simulink model "step4_EvapCompCondHarness"  (R2023a)
settings: Solver=VariableStepAuto  StartTime=0.0  StopTime=36000  RelTol=1e-3  AbsTol=1e-3
model workspace (MATLAB code in the model file):
  | evapCompCondParams;
undefined symbols (not defined in the file): a_x_cond, mdot_air_cond, T0
libraries: fl_lib x43, nesl_utility x9, SimscapeFluids_lib x4
CloseFcn:
  | try,close(h1_step4_EvapCompCondHarness),end
  | clear h1_step4_EvapCompCondHarness
  | try,close(h2_step4_EvapCompCondHarness),end
  | clear h2_step4_EvapCompCondHarness
  | try,close(h3_step4_EvapCompCondHarness),end
  | clear h3_step4_EvapCompCondHarness
  | try,close(h4_step4_EvapCompCondHarness),end
  | clear h4_step4_EvapCompCondHarness
  | 
  | 
  | clear simlog_step4_EvapCompCondHarness
  | clear logsout_step4_EvapCompCondHarness
settings Model: Creator=emcgarri  LastModifiedBy=esmithzb
settings SolverCC: AutoScaleAbsTol=off  AlgebraicLoopSolver=TrustRegion  DecoupledContinuousIntegration=on  MinimalZcImpactIntegration=on  MaxZcPerStep=1
settings DataIOCC: MaxDataPoints=10000  SignalLoggingName=logsout_step4_EvapCompCondHarness
settings OptimizationCC: ReuseModelBlockBuffer=off
settings DebuggingCC: UnconnectedInputMsg=warning  UnconnectedOutputMsg=warning  UnconnectedLineMsg=warning  SymbolicDimsDataTypeCodeGenerationDiagnostic=none
settings ModelReferenceCC: EnableRefExpFcnMdlSchedulingChecks=on
settings SFSimCC: CustomCodeUndefinedFunction=UseInterfaceOnly
settings RTWCC: DLArmComputeVersion=19.05
settings SimscapeCC: SimscapeLogType=all  SimscapeLogSimulationStatistics=on  SimscapeLogOpenViewer=on  SimscapeLogName=simlog_step4_EvapCompCondHarness  SimscapeLogDataHistory=10000

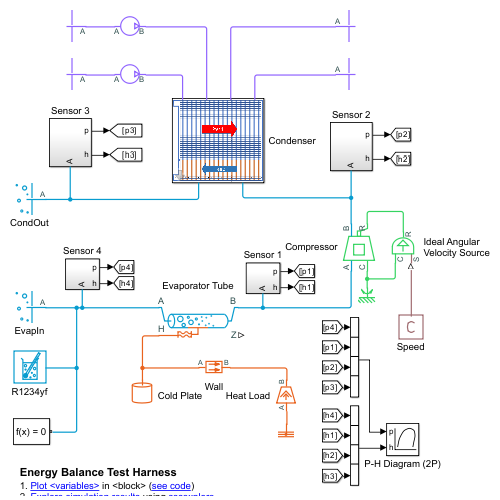
[thumbnail: Simulink's stored preview of the top-level diagram]
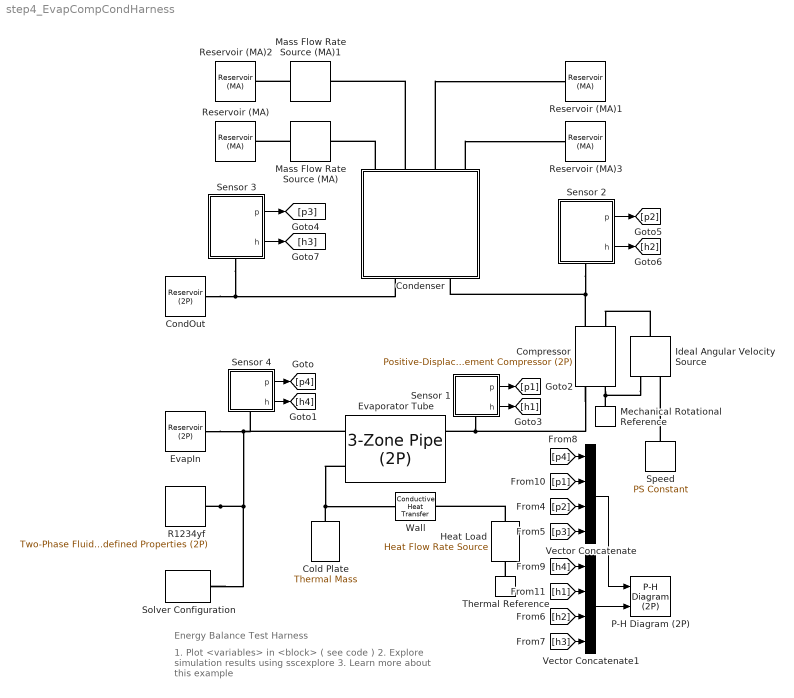
== system step4_EvapCompCondHarness ==
  note: Energy Balance Test Harness
  note: 1. Plot <variables> in <block> ( see code )
      | 2. Explore simulation results using sscexplore
      | 3. Learn more about this example
  Cold Plate : fl_lib/Thermal/Thermal Elements/Thermal Mass  mass_type=foundation.enum.constant_variable.constant  mass=m_plate kg  sp_heat=cp_plate J/(K*kg)  mass_min=1e-6 kg  num_ports=foundation.enum.numPorts2.one  m_specify=off  m_priority=High  m=1 kg  m_nominal_specify=off  m_nominal_unit=kg  m_nominal_value=1  T_specify=on  T_priority=High  T=T0 K  T_nominal_specify=off  T_nominal_unit=K  T_nominal_value=1  Q_specify=off  Q_priority=None  Q=0 W  Q_nominal_specify=off  Q_nominal_unit=W  Q_nominal_value=1
  Compressor : SimscapeFluids_lib/Two-Phase Fluid/Fluid Machines/Positive-Displacement Compressor (2P)  dispSpec=fluids.two_phase_fluid.fluid_machines.enum.DisplacementSpecification.FlowSpeed  v_disp=130 cm^3/rev  mdot_nom=mdot_comp kg/s  omega_nom=N_comp rpm  efficiencySpec=fluids.two_phase_fluid.fluid_machines.enum.VolumetricEfficiencyParameterization.Analytical  eta_nom=eta_v  pr_TLU=[2, 4, 6, 8]  omega_TLU=[800, 1500, 2800, 3300, 4000] rpm  eta_TLU=[.95, .9, .85, .8, .75; .925, .875, .825, .775, .725; .875, .825, .775, .725, .675; .75, .7, .65, .6, .55]  nominalSpec=fluids.two_phase_fluid.fluid_machines.enum.NominalConditionsSpecification.NominalEffandPR  pr_nom=pr_nom  p_in_nom=p_nom_in kPa  T_in_nom=T_nom_in K  T_evap_nom=373.15 K  T_cond_nom=398.15 K  delta_T_nom=10 deltaK  n=gamma1234yf  mechanical_efficiency=eta_m  area_A=a_evap cm^2  area_B=a_cond cm^2  VaporCheck=simscape.enum.assert.action.warn
      settings: InternalSimscapePortConfiguration="{\"Bottom\":[],\"Left\":[{\"id\":\"A\",\"label\":\"A\",\"type\":\"foundation.two_phase_fluid.two_phase_fluid\"},{\"id\":\"C\",\"label\":\"C\",\"type\":\"foundation.mechanical.rotational.rotational\"}],\"Right\":[{\"id\":\"B\",\"label\":\"B\",\"type\":\"foundation.two_phase_fluid.two_phase_fluid\"},{\"id\":\"R\",\"label\":\"R\",\"type\":\"foundation.mechanical.rotational.rotational\"}],\"Top\":[]}"
  CondOut : fl_lib/Two-Phase Fluid/Elements/Reservoir (2P)  pressure_spec=foundation.enum.ReservoirPressureSpec2P.Specified  reservoir_pressure=p0_cond kPa  reservoir_condensing_temperature=373.15 K  reservoir_evaporating_temperature=373.15 K  energy_spec=foundation.enum.ReservoirEnergySpec2P.Enthalpy  reservoir_temperature=293.15 K  reservoir_quality=0.5  reservoir_void_fraction=0.5  reservoir_enthalpy=h0_cond kJ/kg  reservoir_internal_energy=1500 kJ/kg  reservoir_subcooling=5 deltaK  reservoir_superheating=5 deltaK  area_A=a_cond cm^2
  Condenser : Subsystem  ReferencedSubsystem=Condenser_2Pass  p_init=p0_cond kPa  IC_spec=Specific Enthalpy  h_init=h0_cond kJ/kg  x_init=x0  energy_spec=foundation.enum.energy_spec.enthalpy
  EvapIn : fl_lib/Two-Phase Fluid/Elements/Reservoir (2P)  pressure_spec=foundation.enum.ReservoirPressureSpec2P.Specified  reservoir_pressure=p0_evap kPa  reservoir_condensing_temperature=373.15 K  reservoir_evaporating_temperature=373.15 K  energy_spec=foundation.enum.ReservoirEnergySpec2P.Enthalpy  reservoir_temperature=293.15 K  reservoir_quality=0.5  reservoir_void_fraction=0.5  reservoir_enthalpy=h0_evap kJ/kg  reservoir_internal_energy=1500 kJ/kg  reservoir_subcooling=5 deltaK  reservoir_superheating=5 deltaK  area_A=a_evap cm^2
  Evaporator Tube : SimscapeFluids_lib/Two-Phase Fluid/Pipes & Fittings/3-Zone Pipe (2P)  length=l_evap m  area=a_evap cm^2  Dh=d_evap cm  length_add=0 m  roughness=15e-6 m  Re_lam=2000  Re_tur=4000  shape_factor=64  hc_ext=inf W/(m^2*K)  wall_thickness=1 mm  k_wall=k_plate W/(m*K)  c_wall=cp_plate J/(K*kg)  rho_wall=rho_plate kg/m^3  fin_ratio_ext=0  eta_fin_ext=0.5  fin_ratio_int=0  eta_fin_int=0.5  heat_coeff_spec=fluids.two_phase_fluid.pipes_fittings.enum.HeatCoeffSpec.GnielinskiCavalliniZecchin  colburn_coeff_liq=[.023, .8, .33]  colburn_coeff_mix=[.05, .8, .33]  colburn_coeff_vap=[.023, .8, .33]  Nu_lam=3.66  energy_spec=foundation.enum.energy_spec.enthalpy  p_init=p0_evap kPa  T_init=293.15 K  x_init=0.5  alpha_init=0.5  h_init=h0_evap kJ/kg  u_init=1500 kJ/kg
      settings: InternalSimscapePortConfiguration="{\"Bottom\":[],\"Left\":[{\"id\":\"A\",\"label\":\"A\",\"type\":\"foundation.two_phase_fluid.two_phase_fluid\"},{\"id\":\"H\",\"label\":\"H\",\"type\":\"foundation.thermal.thermal\"}],\"Right\":[{\"id\":\"B\",\"label\":\"B\",\"type\":\"foundation.two_phase_fluid.two_phase_fluid\"},{\"id\":\"Z\",\"label\":\"Z\",\"type\":\"output\"}],\"Top\":[]}"
  Heat Load : fl_lib/Thermal/Thermal Sources/Heat Flow Rate Source  heat_flow=1 kW
      settings: InternalSimscapePortConfiguration="{\"Bottom\":[],\"Left\":[{\"id\":\"B\",\"label\":\"B\",\"type\":\"foundation.thermal.thermal\"}],\"Right\":[{\"id\":\"A\",\"label\":\"A\",\"type\":\"foundation.thermal.thermal\"}],\"Top\":[]}"
  Ideal Angular Velocity Source : fl_lib/Mechanical/Mechanical Sources/Ideal Angular Velocity Source
  Mass Flow Rate Source (MA) : fl_lib/Moist Air/Sources/Mass Flow Rate Source (MA)  power_spec=foundation.enum.power_spec.none  mass_flow=mdot_air_cond(2) kg/s  area_A=a_x_cond(2) m^2  area_B=a_x_cond(2) m^2
      settings: InternalSimscapePortConfiguration="{\"Bottom\":[],\"Left\":[{\"id\":\"A\",\"label\":\"A\",\"type\":\"foundation.moist_air.moist_air\"}],\"Right\":[{\"id\":\"B\",\"label\":\"B\",\"type\":\"foundation.moist_air.moist_air\"}],\"Top\":[]}"
  Mass Flow Rate Source (MA)1 : fl_lib/Moist Air/Sources/Mass Flow Rate Source (MA)  power_spec=foundation.enum.power_spec.none  mass_flow=mdot_air_cond(1) kg/s  area_A=a_x_cond(1) cm^2  area_B=a_x_cond(1) cm^2
      settings: InternalSimscapePortConfiguration="{\"Bottom\":[],\"Left\":[{\"id\":\"A\",\"label\":\"A\",\"type\":\"foundation.moist_air.moist_air\"}],\"Right\":[{\"id\":\"B\",\"label\":\"B\",\"type\":\"foundation.moist_air.moist_air\"}],\"Top\":[]}"
  Mechanical Rotational Reference : fl_lib/Mechanical/Rotational Elements/Mechanical Rotational Reference
  P-H Diagram (2P) : SimscapeFluids_lib/Two-Phase Fluid/Utilities/P-H Diagram (2P)
  R1234yf : SimscapeFluids_lib/Two-Phase Fluid/Utilities/Two-Phase Fluid Predefined Properties (2P)  fluid=fluids.two_phase_fluid.utilities.enum.Fluid.R1234yf  p_atm=0.101325 MPa  properties_range_check=simscape.enum.assert.action.error  q_rev=0.01 Pa
  Reservoir (MA) : fl_lib/Moist Air/Elements/Reservoir (MA)  pressure_spec=foundation.enum.pressure_spec.atmospheric  reservoir_pressure=0.101325 MPa  temperature_spec=foundation.enum.temperature_spec.specified  reservoir_temperature=T_air_cond degC  moisture_spec=foundation.enum.moisture_spec.relative_humidity  reservoir_RH=0.5  reservoir_x_w=0.01  reservoir_y_w=0.01  reservoir_HR=0.01  reservoir_Tw=287 K  trace_gas_spec=foundation.enum.trace_gas_spec.mass_fraction  reservoir_x_g=0.00  reservoir_y_g=0.001  RH_ws=1  area_A=a_x_cond(2) cm^2
  Reservoir (MA)1 : fl_lib/Moist Air/Elements/Reservoir (MA)  pressure_spec=foundation.enum.pressure_spec.atmospheric  reservoir_pressure=0.101325 MPa  temperature_spec=foundation.enum.temperature_spec.atmospheric  reservoir_temperature=293.15 K  moisture_spec=foundation.enum.moisture_spec.relative_humidity  reservoir_RH=0.5  reservoir_x_w=0.01  reservoir_y_w=0.01  reservoir_HR=0.01  reservoir_Tw=287 K  trace_gas_spec=foundation.enum.trace_gas_spec.mass_fraction  reservoir_x_g=0.001  reservoir_y_g=0.001  RH_ws=1  area_A=a_x_cond(2) cm^2
  Reservoir (MA)2 : fl_lib/Moist Air/Elements/Reservoir (MA)  pressure_spec=foundation.enum.pressure_spec.atmospheric  reservoir_pressure=0.101325 MPa  temperature_spec=foundation.enum.temperature_spec.specified  reservoir_temperature=T_air_cond degC  moisture_spec=foundation.enum.moisture_spec.relative_humidity  reservoir_RH=0.5  reservoir_x_w=0.01  reservoir_y_w=0.01  reservoir_HR=0.01  reservoir_Tw=287 K  trace_gas_spec=foundation.enum.trace_gas_spec.mass_fraction  reservoir_x_g=0.00  reservoir_y_g=0.001  RH_ws=1  area_A=a_x_cond(1) cm^2
  Reservoir (MA)3 : fl_lib/Moist Air/Elements/Reservoir (MA)  pressure_spec=foundation.enum.pressure_spec.atmospheric  reservoir_pressure=0.101325 MPa  temperature_spec=foundation.enum.temperature_spec.atmospheric  reservoir_temperature=293.15 K  moisture_spec=foundation.enum.moisture_spec.relative_humidity  reservoir_RH=0.5  reservoir_x_w=0.01  reservoir_y_w=0.01  reservoir_HR=0.01  reservoir_Tw=287 K  trace_gas_spec=foundation.enum.trace_gas_spec.mass_fraction  reservoir_x_g=0.001  reservoir_y_g=0.001  RH_ws=1  area_A=a_x_cond(1) cm^2
  Sensor 1 : Subsystem
      settings: PortSchema="{\"entries\":[{\"content\":{\"sides\":[{\"content\":{\"connectorIds\":[]},\"type\":\"ConnectorPlacement.EquallySpacedRectSide\",\"uuid\":\"09a2fde7-9514-415f-ad1a-2358fbc90122\"},{\"content\":{\"connectorIds\":[\"Out1\",\"Out2\"],\"side\":\"RIGHT\"},\"type\":\"ConnectorPlacement.EquallySpacedRectSide\",\"uuid\":\"1a58e595-65c2-481f-a4c6-044a1080df7a\"},{\"content\":{\"connectorIds\":[],\"side\":\"TOP\"},\"type\":\"ConnectorPlacement.EquallySpacedRectSide\",\"uuid\":\"e920d07f-3316-48c2-b5dc-69759bfb2eca\"},{\"content\":{\"connectorIds\":[\"RConn1\"],\"side\":\"BOTTOM\"},\"type\":\"ConnectorPlacement.EquallySpacedRectSide\",\"uuid\":\"ceb1a63b-e9f5-46e4-b72f-4e0e29463411\"}]},\"type\":\"ConnectorPlacement.EquallySpacedConnector\",\"uuid\":\"10759918-f7d5-4efa-b411-b89b519c736f\"}],\"packageUris\":[\"http://schema.mathworks.com/mf0/Connector/R2020b\"],\"version\":\"1.0\"}"
  Sensor 2 : Subsystem
      settings: PortSchema="{\"entries\":[{\"content\":{\"sides\":[{\"content\":{\"connectorIds\":[]},\"type\":\"ConnectorPlacement.EquallySpacedRectSide\",\"uuid\":\"09a2fde7-9514-415f-ad1a-2358fbc90122\"},{\"content\":{\"connectorIds\":[\"Out1\",\"Out2\"],\"side\":\"RIGHT\"},\"type\":\"ConnectorPlacement.EquallySpacedRectSide\",\"uuid\":\"1a58e595-65c2-481f-a4c6-044a1080df7a\"},{\"content\":{\"connectorIds\":[],\"side\":\"TOP\"},\"type\":\"ConnectorPlacement.EquallySpacedRectSide\",\"uuid\":\"e920d07f-3316-48c2-b5dc-69759bfb2eca\"},{\"content\":{\"connectorIds\":[\"RConn1\"],\"side\":\"BOTTOM\"},\"type\":\"ConnectorPlacement.EquallySpacedRectSide\",\"uuid\":\"ceb1a63b-e9f5-46e4-b72f-4e0e29463411\"}]},\"type\":\"ConnectorPlacement.EquallySpacedConnector\",\"uuid\":\"10759918-f7d5-4efa-b411-b89b519c736f\"}],\"packageUris\":[\"http://schema.mathworks.com/mf0/Connector/R2020b\"],\"version\":\"1.0\"}"
  Sensor 3 : Subsystem
      settings: PortSchema="{\"entries\":[{\"content\":{\"sides\":[{\"content\":{\"connectorIds\":[]},\"type\":\"ConnectorPlacement.EquallySpacedRectSide\",\"uuid\":\"09a2fde7-9514-415f-ad1a-2358fbc90122\"},{\"content\":{\"connectorIds\":[\"Out1\",\"Out2\"],\"side\":\"RIGHT\"},\"type\":\"ConnectorPlacement.EquallySpacedRectSide\",\"uuid\":\"1a58e595-65c2-481f-a4c6-044a1080df7a\"},{\"content\":{\"connectorIds\":[],\"side\":\"TOP\"},\"type\":\"ConnectorPlacement.EquallySpacedRectSide\",\"uuid\":\"e920d07f-3316-48c2-b5dc-69759bfb2eca\"},{\"content\":{\"connectorIds\":[\"RConn1\"],\"side\":\"BOTTOM\"},\"type\":\"ConnectorPlacement.EquallySpacedRectSide\",\"uuid\":\"ceb1a63b-e9f5-46e4-b72f-4e0e29463411\"}]},\"type\":\"ConnectorPlacement.EquallySpacedConnector\",\"uuid\":\"10759918-f7d5-4efa-b411-b89b519c736f\"}],\"packageUris\":[\"http://schema.mathworks.com/mf0/Connector/R2020b\"],\"version\":\"1.0\"}"
  Sensor 4 : Subsystem
      settings: PortSchema="{\"entries\":[{\"content\":{\"sides\":[{\"content\":{\"connectorIds\":[]},\"type\":\"ConnectorPlacement.EquallySpacedRectSide\",\"uuid\":\"09a2fde7-9514-415f-ad1a-2358fbc90122\"},{\"content\":{\"connectorIds\":[\"Out1\",\"Out2\"],\"side\":\"RIGHT\"},\"type\":\"ConnectorPlacement.EquallySpacedRectSide\",\"uuid\":\"1a58e595-65c2-481f-a4c6-044a1080df7a\"},{\"content\":{\"connectorIds\":[],\"side\":\"TOP\"},\"type\":\"ConnectorPlacement.EquallySpacedRectSide\",\"uuid\":\"e920d07f-3316-48c2-b5dc-69759bfb2eca\"},{\"content\":{\"connectorIds\":[\"RConn1\"],\"side\":\"BOTTOM\"},\"type\":\"ConnectorPlacement.EquallySpacedRectSide\",\"uuid\":\"ceb1a63b-e9f5-46e4-b72f-4e0e29463411\"}]},\"type\":\"ConnectorPlacement.EquallySpacedConnector\",\"uuid\":\"10759918-f7d5-4efa-b411-b89b519c736f\"}],\"packageUris\":[\"http://schema.mathworks.com/mf0/Connector/R2020b\"],\"version\":\"1.0\"}"
  Solver Configuration : nesl_utility/Solver Configuration  PhysicalDomain=network_engine_domain  SubClassName=solver  LeftPortType=input  RightPortType=generic  Tones=[]  Harmonics=[]  SimulateNoise=off  Profile=off  UseLocalSampling=off  EnableSwitchedLinearOptims=on  FrequencyDomain=off  UseCCode=off  RelTol=0.001  AbsTol=1e-06  MinStep=1e-09  ToWorkspace=off  RevertToSquareIcSolve=off  NumHomotopyIterations=100  PhasorMode=off  PhasorModeNumHarmonics=1  ConsistencySolver=NEWTON_XTOL_AFTER_FTOL  IndexReductionMethod=DerivativeReplacement  DoDC=on  ResidualTolerance=1e-09  ConsistencyTolSource=GLOBAL  ConsistencyAbsTol=0.001  ConsistencyRelTol=0.001  ConsistencyTolFactor=0.001  UseLocalSolver=off  LocalSolverChoice=NE_BACKWARD_EULER_ADVANCER  ResolveIndetEquations=on  FunctionEvalNumThread=1  LocalSolverSampleTime=0.001  DoFixedCost=off  MaxNonlinIter=3  MaxModeIter=2  ComputeImpulses=off  ImpulseIterations=2  LinearAlgebra=auto  LinearAlgebraNumThread=0  EquationFormulation=NE_TIME_EF  DelaysMemoryBudget=1024  AutomaticFiltering=off  FilteringTimeConstant=0.001  PartitionStorageMethod=AS_NEEDED  PartitionMemoryBudget=1024  PartitionMethod=ROBUST
  Speed : fl_lib/Physical Signals/Sources/PS Constant  constant=3600 rpm
  Thermal Reference : fl_lib/Thermal/Thermal Elements/Thermal Reference
  Vector Concatenate : Concatenate  NumInputs=4
  Vector Concatenate1 : Concatenate  NumInputs=4
  Wall : fl_lib/Thermal/Thermal Elements/Conductive Heat Transfer  thermal_type=foundation.enum.ConstantVariableTabulated.Constant  wall_geometry=foundation.enum.ConductionWallGeometry.Planar  area=a_plate cm^2  thickness=t_cond_plate cm  d_in=0.05 m  d_out=0.1 m  L=1 m  th_cond_min=10 W/(K*m)  th_cond=k_plate W/(m*K)  th_cond_TLU=[413, 401, 392, 383, 371, 357, 342] W/(K*m)  temp_TLU=[200, 273, 400, 600, 800, 1000, 1200] K  T_specify=off  T_priority=None  T=0 K  T_nominal_specify=off  T_nominal_unit=K  T_nominal_value=1  Q_specify=off  Q_priority=None  Q=0 W  Q_nominal_specify=off  Q_nominal_unit=W  Q_nominal_value=1
  wires:
  Sensor 4/1(p) -> [p4]
  Sensor 4/2(h) -> [h4]
  Sensor 1/1(p) -> [p1]
  Sensor 1/2(h) -> [h1]
  [h4] -> Vector Concatenate1/1
  [h3] -> Vector Concatenate1/4
  [p1] -> Vector Concatenate/2
  [h1] -> Vector Concatenate1/2
  Sensor 3/2(h) -> [h3]
  [h2] -> Vector Concatenate1/3
  Sensor 2/2(h) -> [h2]
  [p2] -> Vector Concatenate/3
  Sensor 3/1(p) -> [p3]
  [p4] -> Vector Concatenate/1
  Sensor 2/1(p) -> [p2]
  [p3] -> Vector Concatenate/4
  Vector Concatenate1/1 -> P-H Diagram (2P)/2
  Vector Concatenate/1 -> P-H Diagram (2P)/1
  connections:
  Cold Plate/LConn1 -- Wall/LConn1 -- Evaporator Tube/LConn2
  Thermal Reference/LConn1 -- Heat Load/RConn1
  Heat Load/LConn1 -- Wall/RConn1
  Mechanical Rotational Reference/LConn1 -- Ideal Angular Velocity Source/RConn2 -- Compressor/LConn2
  Ideal Angular Velocity Source/LConn1 -- Compressor/RConn2
  CondOut/LConn1 -- Condenser/LConn1 -- Sensor 3/RConn1
  R1234yf/RConn1 -- EvapIn/LConn1 -- Evaporator Tube/LConn1 -- Sensor 4/RConn1 -- Solver Configuration/RConn1
  Sensor 1/RConn1 -- Evaporator Tube/RConn1 -- Compressor/LConn1
  Mass Flow Rate Source (MA)/LConn1 -- Reservoir (MA)/LConn1
  Mass Flow Rate Source (MA)1/LConn1 -- Reservoir (MA)2/LConn1
  Condenser/RConn1 -- Mass Flow Rate Source (MA)/RConn1
  Condenser/RConn2 -- Mass Flow Rate Source (MA)1/RConn1
  Condenser/RConn3 -- Reservoir (MA)1/LConn1
  Condenser/RConn4 -- Reservoir (MA)3/LConn1
  Compressor/RConn1 -- Sensor 2/RConn1 -- Condenser/LConn2
  Speed/RConn1 -- Ideal Angular Velocity Source/RConn1

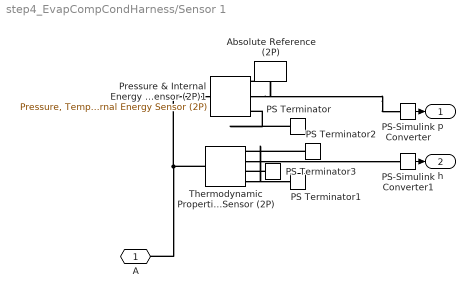
== system step4_EvapCompCondHarness/Sensor 1 ==
  Absolute Reference (2P) : fl_lib/Two-Phase Fluid/Elements/Absolute Reference (2P)
  PS Terminator{,1..3} (4 alike) : fl_lib/Physical Signals/Sinks/PS Terminator
  PS-Simulink Converter : nesl_utility/PS-Simulink Converter  PhysicalDomain=network_engine_domain  SubClassName=ps_output  LeftPortType=input  RightPortType=output  PseudoPeriodic=off  Frequencies=[]  VectorFormat=1-D array  Unit=MPa  AffineConversion=off
  PS-Simulink Converter1 : nesl_utility/PS-Simulink Converter  PhysicalDomain=network_engine_domain  SubClassName=ps_output  LeftPortType=input  RightPortType=output  PseudoPeriodic=off  Frequencies=[]  VectorFormat=1-D array  Unit=kJ/kg  AffineConversion=off
  Pressure & Internal Energy Sensor (2P)1 : fl_lib/Two-Phase Fluid/Sensors/Pressure, Temperature & Internal Energy Sensor (2P)  reference=foundation.enum.MeasurementReference.difference  pressure=true  pressure_spec=foundation.enum.PressureMeasementSpec.Absolute  temperature=false  internal_energy=true
      settings: InternalSimscapePortConfiguration="{\"Bottom\":[{\"id\":\"U\",\"label\":\"U\",\"type\":\"output\"}],\"Left\":[{\"id\":\"A\",\"label\":\"A\",\"type\":\"foundation.two_phase_fluid.two_phase_fluid\"}],\"Right\":[{\"id\":\"B\",\"label\":\"B\",\"type\":\"foundation.two_phase_fluid.two_phase_fluid\"},{\"id\":\"P\",\"label\":\"P\",\"type\":\"output\"}],\"Top\":[]}"
  Thermodynamic Properties Sensor (2P) : fl_lib/Two-Phase Fluid/Sensors/Thermodynamic Properties Sensor (2P)  temperature=true  enthalpy=true  density=false  specific_volume=true  entropy=true
      settings: InternalSimscapePortConfiguration="{\"Bottom\":[{\"id\":\"V\",\"label\":\"v\",\"type\":\"output\"},{\"id\":\"S\",\"label\":\"s\",\"type\":\"output\"}],\"Left\":[{\"id\":\"A\",\"label\":\"A\",\"type\":\"foundation.two_phase_fluid.two_phase_fluid\"}],\"Right\":[{\"id\":\"T\",\"label\":\"T\",\"type\":\"output\"},{\"id\":\"H\",\"label\":\"h\",\"type\":\"output\"}],\"Top\":[]}"
  A : PMIOPort  Side=Right
  p : Outport
  h : Outport  Port=2
  wires:
  PS-Simulink Converter1/1 -> h/1
  PS-Simulink Converter/1 -> p/1
  connections:
  Thermodynamic Properties Sensor (2P)/RConn2 -- PS-Simulink Converter1/LConn1
  PS Terminator3/LConn1 -- Thermodynamic Properties Sensor (2P)/RConn3
  PS Terminator/LConn1 -- Pressure & Internal Energy Sensor (2P)1/RConn3
  Thermodynamic Properties Sensor (2P)/LConn1 -- A/RConn1 -- Pressure & Internal Energy Sensor (2P)1/LConn1
  Thermodynamic Properties Sensor (2P)/RConn4 -- PS Terminator1/LConn1
  PS Terminator2/LConn1 -- Thermodynamic Properties Sensor (2P)/RConn1
  Pressure & Internal Energy Sensor (2P)1/RConn2 -- PS-Simulink Converter/LConn1
  Absolute Reference (2P)/LConn1 -- Pressure & Internal Energy Sensor (2P)1/RConn1

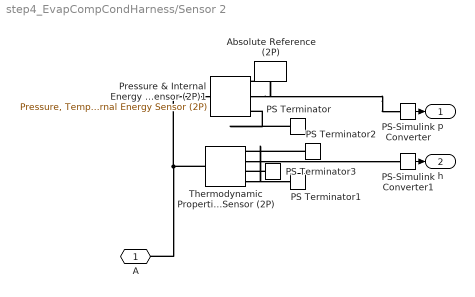
== system step4_EvapCompCondHarness/Sensor 2 ==
  Absolute Reference (2P) : fl_lib/Two-Phase Fluid/Elements/Absolute Reference (2P)
  PS Terminator{,1..3} (4 alike) : fl_lib/Physical Signals/Sinks/PS Terminator
  PS-Simulink Converter : nesl_utility/PS-Simulink Converter  PhysicalDomain=network_engine_domain  SubClassName=ps_output  LeftPortType=input  RightPortType=output  PseudoPeriodic=off  Frequencies=[]  VectorFormat=1-D array  Unit=MPa  AffineConversion=off
  PS-Simulink Converter1 : nesl_utility/PS-Simulink Converter  PhysicalDomain=network_engine_domain  SubClassName=ps_output  LeftPortType=input  RightPortType=output  PseudoPeriodic=off  Frequencies=[]  VectorFormat=1-D array  Unit=kJ/kg  AffineConversion=off
  Pressure & Internal Energy Sensor (2P)1 : fl_lib/Two-Phase Fluid/Sensors/Pressure, Temperature & Internal Energy Sensor (2P)  reference=foundation.enum.MeasurementReference.difference  pressure=true  pressure_spec=foundation.enum.PressureMeasementSpec.Absolute  temperature=false  internal_energy=true
      settings: InternalSimscapePortConfiguration="{\"Bottom\":[{\"id\":\"U\",\"label\":\"U\",\"type\":\"output\"}],\"Left\":[{\"id\":\"A\",\"label\":\"A\",\"type\":\"foundation.two_phase_fluid.two_phase_fluid\"}],\"Right\":[{\"id\":\"B\",\"label\":\"B\",\"type\":\"foundation.two_phase_fluid.two_phase_fluid\"},{\"id\":\"P\",\"label\":\"P\",\"type\":\"output\"}],\"Top\":[]}"
  Thermodynamic Properties Sensor (2P) : fl_lib/Two-Phase Fluid/Sensors/Thermodynamic Properties Sensor (2P)  temperature=true  enthalpy=true  density=false  specific_volume=true  entropy=true
      settings: InternalSimscapePortConfiguration="{\"Bottom\":[{\"id\":\"V\",\"label\":\"v\",\"type\":\"output\"},{\"id\":\"S\",\"label\":\"s\",\"type\":\"output\"}],\"Left\":[{\"id\":\"A\",\"label\":\"A\",\"type\":\"foundation.two_phase_fluid.two_phase_fluid\"}],\"Right\":[{\"id\":\"T\",\"label\":\"T\",\"type\":\"output\"},{\"id\":\"H\",\"label\":\"h\",\"type\":\"output\"}],\"Top\":[]}"
  A : PMIOPort  Side=Right
  p : Outport
  h : Outport  Port=2
  wires:
  PS-Simulink Converter1/1 -> h/1
  PS-Simulink Converter/1 -> p/1
  connections:
  Thermodynamic Properties Sensor (2P)/RConn2 -- PS-Simulink Converter1/LConn1
  PS Terminator3/LConn1 -- Thermodynamic Properties Sensor (2P)/RConn3
  PS Terminator/LConn1 -- Pressure & Internal Energy Sensor (2P)1/RConn3
  Thermodynamic Properties Sensor (2P)/LConn1 -- Pressure & Internal Energy Sensor (2P)1/LConn1 -- A/RConn1
  Thermodynamic Properties Sensor (2P)/RConn4 -- PS Terminator1/LConn1
  PS Terminator2/LConn1 -- Thermodynamic Properties Sensor (2P)/RConn1
  Pressure & Internal Energy Sensor (2P)1/RConn2 -- PS-Simulink Converter/LConn1
  Absolute Reference (2P)/LConn1 -- Pressure & Internal Energy Sensor (2P)1/RConn1

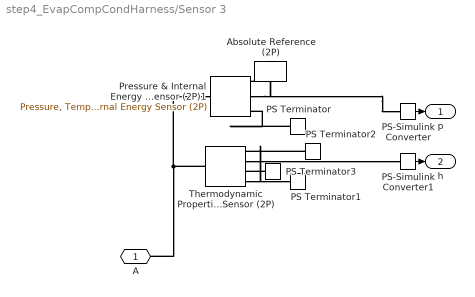
== system step4_EvapCompCondHarness/Sensor 3 ==
  Absolute Reference (2P) : fl_lib/Two-Phase Fluid/Elements/Absolute Reference (2P)
  PS Terminator{,1..3} (4 alike) : fl_lib/Physical Signals/Sinks/PS Terminator
  PS-Simulink Converter : nesl_utility/PS-Simulink Converter  PhysicalDomain=network_engine_domain  SubClassName=ps_output  LeftPortType=input  RightPortType=output  PseudoPeriodic=off  Frequencies=[]  VectorFormat=1-D array  Unit=MPa  AffineConversion=off
  PS-Simulink Converter1 : nesl_utility/PS-Simulink Converter  PhysicalDomain=network_engine_domain  SubClassName=ps_output  LeftPortType=input  RightPortType=output  PseudoPeriodic=off  Frequencies=[]  VectorFormat=1-D array  Unit=kJ/kg  AffineConversion=off
  Pressure & Internal Energy Sensor (2P)1 : fl_lib/Two-Phase Fluid/Sensors/Pressure, Temperature & Internal Energy Sensor (2P)  reference=foundation.enum.MeasurementReference.difference  pressure=true  pressure_spec=foundation.enum.PressureMeasementSpec.Absolute  temperature=false  internal_energy=true
      settings: InternalSimscapePortConfiguration="{\"Bottom\":[{\"id\":\"U\",\"label\":\"U\",\"type\":\"output\"}],\"Left\":[{\"id\":\"A\",\"label\":\"A\",\"type\":\"foundation.two_phase_fluid.two_phase_fluid\"}],\"Right\":[{\"id\":\"B\",\"label\":\"B\",\"type\":\"foundation.two_phase_fluid.two_phase_fluid\"},{\"id\":\"P\",\"label\":\"P\",\"type\":\"output\"}],\"Top\":[]}"
  Thermodynamic Properties Sensor (2P) : fl_lib/Two-Phase Fluid/Sensors/Thermodynamic Properties Sensor (2P)  temperature=true  enthalpy=true  density=false  specific_volume=true  entropy=true
      settings: InternalSimscapePortConfiguration="{\"Bottom\":[{\"id\":\"V\",\"label\":\"v\",\"type\":\"output\"},{\"id\":\"S\",\"label\":\"s\",\"type\":\"output\"}],\"Left\":[{\"id\":\"A\",\"label\":\"A\",\"type\":\"foundation.two_phase_fluid.two_phase_fluid\"}],\"Right\":[{\"id\":\"T\",\"label\":\"T\",\"type\":\"output\"},{\"id\":\"H\",\"label\":\"h\",\"type\":\"output\"}],\"Top\":[]}"
  A : PMIOPort  Side=Right
  p : Outport
  h : Outport  Port=2
  wires:
  PS-Simulink Converter1/1 -> h/1
  PS-Simulink Converter/1 -> p/1
  connections:
  Thermodynamic Properties Sensor (2P)/RConn2 -- PS-Simulink Converter1/LConn1
  PS Terminator3/LConn1 -- Thermodynamic Properties Sensor (2P)/RConn3
  PS Terminator/LConn1 -- Pressure & Internal Energy Sensor (2P)1/RConn3
  Thermodynamic Properties Sensor (2P)/LConn1 -- Pressure & Internal Energy Sensor (2P)1/LConn1 -- A/RConn1
  Thermodynamic Properties Sensor (2P)/RConn4 -- PS Terminator1/LConn1
  PS Terminator2/LConn1 -- Thermodynamic Properties Sensor (2P)/RConn1
  Pressure & Internal Energy Sensor (2P)1/RConn2 -- PS-Simulink Converter/LConn1
  Absolute Reference (2P)/LConn1 -- Pressure & Internal Energy Sensor (2P)1/RConn1

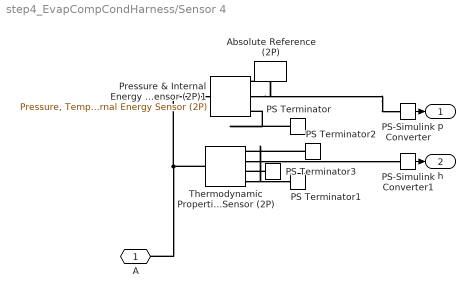
== system step4_EvapCompCondHarness/Sensor 4 ==
  Absolute Reference (2P) : fl_lib/Two-Phase Fluid/Elements/Absolute Reference (2P)
  PS Terminator{,1..3} (4 alike) : fl_lib/Physical Signals/Sinks/PS Terminator
  PS-Simulink Converter : nesl_utility/PS-Simulink Converter  PhysicalDomain=network_engine_domain  SubClassName=ps_output  LeftPortType=input  RightPortType=output  PseudoPeriodic=off  Frequencies=[]  VectorFormat=1-D array  Unit=MPa  AffineConversion=off
  PS-Simulink Converter1 : nesl_utility/PS-Simulink Converter  PhysicalDomain=network_engine_domain  SubClassName=ps_output  LeftPortType=input  RightPortType=output  PseudoPeriodic=off  Frequencies=[]  VectorFormat=1-D array  Unit=kJ/kg  AffineConversion=off
  Pressure & Internal Energy Sensor (2P)1 : fl_lib/Two-Phase Fluid/Sensors/Pressure, Temperature & Internal Energy Sensor (2P)  reference=foundation.enum.MeasurementReference.difference  pressure=true  pressure_spec=foundation.enum.PressureMeasementSpec.Absolute  temperature=false  internal_energy=true
      settings: InternalSimscapePortConfiguration="{\"Bottom\":[{\"id\":\"U\",\"label\":\"U\",\"type\":\"output\"}],\"Left\":[{\"id\":\"A\",\"label\":\"A\",\"type\":\"foundation.two_phase_fluid.two_phase_fluid\"}],\"Right\":[{\"id\":\"B\",\"label\":\"B\",\"type\":\"foundation.two_phase_fluid.two_phase_fluid\"},{\"id\":\"P\",\"label\":\"P\",\"type\":\"output\"}],\"Top\":[]}"
  Thermodynamic Properties Sensor (2P) : fl_lib/Two-Phase Fluid/Sensors/Thermodynamic Properties Sensor (2P)  temperature=true  enthalpy=true  density=false  specific_volume=true  entropy=true
      settings: InternalSimscapePortConfiguration="{\"Bottom\":[{\"id\":\"V\",\"label\":\"v\",\"type\":\"output\"},{\"id\":\"S\",\"label\":\"s\",\"type\":\"output\"}],\"Left\":[{\"id\":\"A\",\"label\":\"A\",\"type\":\"foundation.two_phase_fluid.two_phase_fluid\"}],\"Right\":[{\"id\":\"T\",\"label\":\"T\",\"type\":\"output\"},{\"id\":\"H\",\"label\":\"h\",\"type\":\"output\"}],\"Top\":[]}"
  A : PMIOPort  Side=Right
  p : Outport
  h : Outport  Port=2
  wires:
  PS-Simulink Converter1/1 -> h/1
  PS-Simulink Converter/1 -> p/1
  connections:
  Thermodynamic Properties Sensor (2P)/RConn2 -- PS-Simulink Converter1/LConn1
  PS Terminator3/LConn1 -- Thermodynamic Properties Sensor (2P)/RConn3
  PS Terminator/LConn1 -- Pressure & Internal Energy Sensor (2P)1/RConn3
  Thermodynamic Properties Sensor (2P)/LConn1 -- Pressure & Internal Energy Sensor (2P)1/LConn1 -- A/RConn1
  Thermodynamic Properties Sensor (2P)/RConn4 -- PS Terminator1/LConn1
  PS Terminator2/LConn1 -- Thermodynamic Properties Sensor (2P)/RConn1
  Pressure & Internal Energy Sensor (2P)1/RConn2 -- PS-Simulink Converter/LConn1
  Absolute Reference (2P)/LConn1 -- Pressure & Internal Energy Sensor (2P)1/RConn1
